simulink model "BMS"  (R2024b)
settings: Solver=ode23tb  StartTime=0.0  StopTime=1  RelTol=1e-3  EnableMultiTasking=on
PreLoadFcn:
  | % Data of Solar Panel
  | %5000[W]/130[W]
  | % Total power generated by solar panel reaches 5[KW].
  | % each solar panel generates power 130[kW].
  | V = [0    40 80 120 160 180 200 217 240 260 280];
  | I = 5000/130*[0.68 0.675 0.67 0.665 0.660 0.655 0.640 0.6 0.48 0.28 0];
  | 
  | %subplot(211);plot(V,I);xlabel('Voltage[V]');ylabel('Current[a]')
  | %subplot(212);plot(V.*I);title('Power[W]')
  | 
  | % Sample Time[s]
  | Ts =5e-6;
  | 
  | 
  | %MPPT + PV Control
  | % PI control pamameter of Voltage control(Outer loop)
  | Kp_V = 50e-3;
  | Ki_V = 10;
  | 
  | % PI Control pamameter of Current control(Inner loop)
  | Kp_I = 25e-3;
  | Ki_I = 10;
  | 
  | % Utility Interconnection Control
  | % PI Control pamameter of Voltage control(Outer loop)
  | Kp_V2 = 0.01;
  | Ki_V2 = 25;
  | 
  | % PI control pamameter of Current control(Inner loop)
  | Kp_I2 = 0.01;
  | Ki_I2 = 25;
  | 
  | 
  | % Difference of voltege using in MPPT
  | dV = 0.5;
  | 
  | % Battery Control
  | % PI Control pamameter of Voltage control(Outer loop)
  | Kp_VB = 0.4;
  | Ki_VB = 2;
  | 
  | % PI control pamameter of Current control(Inner loop)
  | Kp_IB = 0.1;
  | Ki_IB = 0.5;
undefined symbols (not defined in the file): Acid, Ion, Lead, Lithium, sigbuilder_block
libraries: spsBreakerLib x120, spsBatteryLib x111, spsSeriesRLCBranchLib x59, spsVoltageMeasurementLib x17, spsIdealSwitchLib x15, spsMosfetLib x11, slpidlib x9, spsCurrentMeasurementLib x7, spsPWMGeneratorDCDCLib x7, spsDiodeLib x6, spsPWMGenerator2LevelLib x5, spspowerguiLib x3
(part 3 of 6)

== system BMS/Subsystem18/Subsystem7 ==
  Battery : spsBatteryLib/Battery  BatType=Lithium-Ion  NomV=12  NomQ=10  SOC=95  Batt_Tr=30  PresetModel=on  MaxQ=10  MinV=9  FullV=13.9678  Dis_rate=4.3478  R=0.012  Normal_OP=9.0435  expZone="[12.9646     0.491304]"
  Breaker{,1..3} (4 alike) : spsBreakerLib/Breaker  InitialState=0  SwitchingTimes="[1/60  5/60]"  External=on  BreakerResistance=0.01  SnubberResistance=1e6  SnubberCapacitance=inf  Measurements=None  MoreParameters=on  NoBreakLoop=off
  Bus Selector : BusSelector  OutputSignals=SOC (%),Current (A),Voltage (V)
  Scope : Scope  NumInputPorts=3
  Series RLC Branch : spsSeriesRLCBranchLib/Series RLC Branch  LConnTagsString=__new0  RConnTagsString=__new0  BranchType=R  Resistance=1  Inductance=1e-3  SetiL0=off  InitialCurrent=0  Capacitance=1e-6  Setx0=off  InitialVoltage=0  Measurements=None
  + : PMIOPort  Side=Right
  - : PMIOPort  Port=2  Side=Right
  tag scope: s11=global
  wires:
  Battery/1 -> Bus Selector/1
  [c11] -> Breaker3/1, Breaker/1
  Bus Selector/2 -> Scope/2  "<Current (A)>"
  [d11] -> Breaker1/1, Breaker2/1
  Bus Selector/3 -> Scope/3  "<Voltage (V)>"
  Bus Selector/1 -> [s11], Scope/1  "<SOC (%)>"
  connections:
  Breaker2/LConn1 -- Breaker3/RConn1 -- Battery/LConn2
  Breaker1/LConn1 -- Battery/LConn1 -- Breaker/RConn1
  +/RConn1 -- Breaker/LConn1
  Series RLC Branch/LConn1 -- Breaker2/RConn1
  Series RLC Branch/RConn1 -- Breaker1/RConn1
  -/RConn1 -- Breaker3/LConn1

== system BMS/Subsystem18/Subsystem8 ==
  Battery : spsBatteryLib/Battery  BatType=Lithium-Ion  NomV=12  NomQ=10  SOC=95  Batt_Tr=30  PresetModel=on  MaxQ=10  MinV=9  FullV=13.9678  Dis_rate=4.3478  R=0.012  Normal_OP=9.0435  expZone="[12.9646     0.491304]"
  Breaker{,1..3} (4 alike) : spsBreakerLib/Breaker  InitialState=0  SwitchingTimes="[1/60  5/60]"  External=on  BreakerResistance=0.01  SnubberResistance=1e6  SnubberCapacitance=inf  Measurements=None  MoreParameters=on  NoBreakLoop=off
  Bus Selector : BusSelector  OutputSignals=SOC (%),Current (A),Voltage (V)
  Scope : Scope  NumInputPorts=3
  Series RLC Branch : spsSeriesRLCBranchLib/Series RLC Branch  LConnTagsString=__new0  RConnTagsString=__new0  BranchType=R  Resistance=1  Inductance=1e-3  SetiL0=off  InitialCurrent=0  Capacitance=1e-6  Setx0=off  InitialVoltage=0  Measurements=None
  + : PMIOPort  Side=Right
  - : PMIOPort  Port=2  Side=Right
  tag scope: s19=global
  wires:
  Battery/1 -> Bus Selector/1
  [c19] -> Breaker3/1, Breaker/1
  Bus Selector/2 -> Scope/2  "<Current (A)>"
  [d19] -> Breaker1/1, Breaker2/1
  Bus Selector/3 -> Scope/3  "<Voltage (V)>"
  Bus Selector/1 -> [s19], Scope/1  "<SOC (%)>"
  connections:
  Breaker2/LConn1 -- Breaker3/RConn1 -- Battery/LConn2
  Breaker1/LConn1 -- Battery/LConn1 -- Breaker/RConn1
  +/RConn1 -- Breaker/LConn1
  Series RLC Branch/LConn1 -- Breaker2/RConn1
  Series RLC Branch/RConn1 -- Breaker1/RConn1
  -/RConn1 -- Breaker3/LConn1

== system BMS/Subsystem18/Subsystem9 ==
  Battery : spsBatteryLib/Battery  BatType=Lithium-Ion  NomV=12  NomQ=10  SOC=95  Batt_Tr=30  PresetModel=on  MaxQ=10  MinV=9  FullV=13.9678  Dis_rate=4.3478  R=0.012  Normal_OP=9.0435  expZone="[12.9646     0.491304]"
  Breaker{,1..3} (4 alike) : spsBreakerLib/Breaker  InitialState=0  SwitchingTimes="[1/60  5/60]"  External=on  BreakerResistance=0.01  SnubberResistance=1e6  SnubberCapacitance=inf  Measurements=None  MoreParameters=on  NoBreakLoop=off
  Bus Selector : BusSelector  OutputSignals=SOC (%),Current (A),Voltage (V)
  Scope : Scope  NumInputPorts=3
  Series RLC Branch : spsSeriesRLCBranchLib/Series RLC Branch  LConnTagsString=__new0  RConnTagsString=__new0  BranchType=R  Resistance=1  Inductance=1e-3  SetiL0=off  InitialCurrent=0  Capacitance=1e-6  Setx0=off  InitialVoltage=0  Measurements=None
  + : PMIOPort  Side=Right
  - : PMIOPort  Port=2  Side=Right
  tag scope: s20=global
  wires:
  Battery/1 -> Bus Selector/1
  [c20] -> Breaker3/1, Breaker/1
  Bus Selector/2 -> Scope/2  "<Current (A)>"
  [d20] -> Breaker1/1, Breaker2/1
  Bus Selector/3 -> Scope/3  "<Voltage (V)>"
  Bus Selector/1 -> [s20], Scope/1  "<SOC (%)>"
  connections:
  Breaker2/LConn1 -- Breaker3/RConn1 -- Battery/LConn2
  Breaker1/LConn1 -- Battery/LConn1 -- Breaker/RConn1
  +/RConn1 -- Breaker/LConn1
  Series RLC Branch/LConn1 -- Breaker2/RConn1
  Series RLC Branch/RConn1 -- Breaker1/RConn1
  -/RConn1 -- Breaker3/LConn1

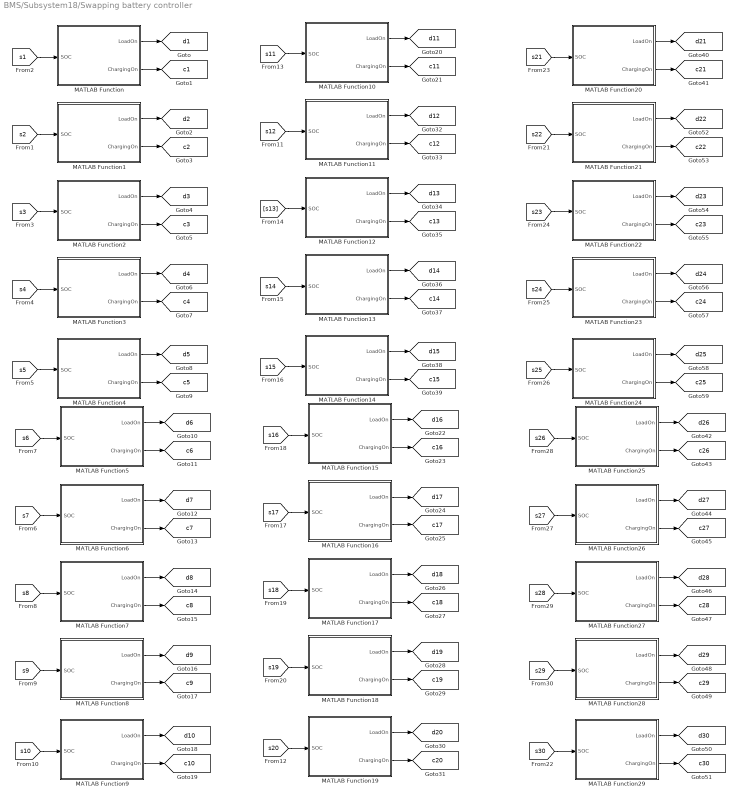
== system BMS/Subsystem18/Swapping battery controller ==
  MATLAB Function : MATLAB Function  TreatAsAtomicUnit=on
  MATLAB Function1 : MATLAB Function  TreatAsAtomicUnit=on
  MATLAB Function10 : MATLAB Function  TreatAsAtomicUnit=on
  MATLAB Function11 : MATLAB Function  TreatAsAtomicUnit=on
  MATLAB Function12 : MATLAB Function  TreatAsAtomicUnit=on
  MATLAB Function13 : MATLAB Function  TreatAsAtomicUnit=on
  MATLAB Function14 : MATLAB Function  TreatAsAtomicUnit=on
  MATLAB Function15 : MATLAB Function  TreatAsAtomicUnit=on
  MATLAB Function16 : MATLAB Function  TreatAsAtomicUnit=on
  MATLAB Function17 : MATLAB Function  TreatAsAtomicUnit=on
  MATLAB Function18 : MATLAB Function  TreatAsAtomicUnit=on
  MATLAB Function19 : MATLAB Function  TreatAsAtomicUnit=on
  MATLAB Function2 : MATLAB Function  TreatAsAtomicUnit=on
  MATLAB Function20 : MATLAB Function  TreatAsAtomicUnit=on
  MATLAB Function21 : MATLAB Function  TreatAsAtomicUnit=on
  MATLAB Function22 : MATLAB Function  TreatAsAtomicUnit=on
  MATLAB Function23 : MATLAB Function  TreatAsAtomicUnit=on
  MATLAB Function24 : MATLAB Function  TreatAsAtomicUnit=on
  MATLAB Function25 : MATLAB Function  TreatAsAtomicUnit=on
  MATLAB Function26 : MATLAB Function  TreatAsAtomicUnit=on
  MATLAB Function27 : MATLAB Function  TreatAsAtomicUnit=on
  MATLAB Function28 : MATLAB Function  TreatAsAtomicUnit=on
  MATLAB Function29 : MATLAB Function  TreatAsAtomicUnit=on
  MATLAB Function3 : MATLAB Function  TreatAsAtomicUnit=on
  MATLAB Function4 : MATLAB Function  TreatAsAtomicUnit=on
  MATLAB Function5 : MATLAB Function  TreatAsAtomicUnit=on
  MATLAB Function6 : MATLAB Function  TreatAsAtomicUnit=on
  MATLAB Function7 : MATLAB Function  TreatAsAtomicUnit=on
  MATLAB Function8 : MATLAB Function  TreatAsAtomicUnit=on
  MATLAB Function9 : MATLAB Function  TreatAsAtomicUnit=on
  tag scope: c10=global, c11=global, c12=global, c13=global, c14=global, c15=global, c16=global, c17=global, c18=global, c19=global, c1=global, c20=global, c21=global, c22=global, c23=global, c24=global, c25=global, c26=global, c27=global, c28=global, c29=global, c2=global, c30=global, c3=global, c4=global, c5=global, c6=global, c7=global, c8=global, c9=global, d10=global, d11=global, d12=global, d13=global, d14=global, d15=global, d16=global, d17=global, d18=global, d19=global, d1=global, d20=global, d21=global, d22=global, d23=global, d24=global, d25=global, d26=global, d27=global, d28=global, d29=global, d2=global, d30=global, d3=global, d4=global, d5=global, d6=global, d7=global, d8=global, d9=global
  wires:
  MATLAB Function10/1(LoadOn) -> [d11]
  MATLAB Function1/2(ChargingOn) -> [c2]
  [s20] -> MATLAB Function19/1(SOC)
  [s22] -> MATLAB Function21/1(SOC)
  MATLAB Function5/1(LoadOn) -> [d6]
  [s16] -> MATLAB Function15/1(SOC)
  [s5] -> MATLAB Function4/1(SOC)
  MATLAB Function/2(ChargingOn) -> [c1]
  MATLAB Function2/2(ChargingOn) -> [c3]
  MATLAB Function26/1(LoadOn) -> [d27]
  [s21] -> MATLAB Function20/1(SOC)
  MATLAB Function18/1(LoadOn) -> [d19]
  MATLAB Function7/2(ChargingOn) -> [c8]
  MATLAB Function12/2(ChargingOn) -> [c13]
  MATLAB Function28/1(LoadOn) -> [d29]
  MATLAB Function4/2(ChargingOn) -> [c5]
  MATLAB Function25/2(ChargingOn) -> [c26]
  [s1] -> MATLAB Function/1(SOC)
  MATLAB Function11/2(ChargingOn) -> [c12]
  MATLAB Function/1(LoadOn) -> [d1]
  MATLAB Function16/1(LoadOn) -> [d17]
  MATLAB Function10/2(ChargingOn) -> [c11]
  [s15] -> MATLAB Function14/1(SOC)
  [s12] -> MATLAB Function11/1(SOC)
  [s3] -> MATLAB Function2/1(SOC)
  MATLAB Function2/1(LoadOn) -> [d3]
  MATLAB Function17/1(LoadOn) -> [d18]
  MATLAB Function13/2(ChargingOn) -> [c14]
  MATLAB Function4/1(LoadOn) -> [d5]
  MATLAB Function14/2(ChargingOn) -> [c15]
  MATLAB Function3/1(LoadOn) -> [d4]
  MATLAB Function6/2(ChargingOn) -> [c7]
  [s7] -> MATLAB Function6/1(SOC)
  MATLAB Function15/1(LoadOn) -> [d16]
  MATLAB Function26/2(ChargingOn) -> [c27]
  [s8] -> MATLAB Function7/1(SOC)
  MATLAB Function6/1(LoadOn) -> [d7]
  MATLAB Function13/1(LoadOn) -> [d14]
  MATLAB Function16/2(ChargingOn) -> [c17]
  MATLAB Function18/2(ChargingOn) -> [c19]
  MATLAB Function5/2(ChargingOn) -> [c6]
  [s6] -> MATLAB Function5/1(SOC)
  [s18] -> MATLAB Function17/1(SOC)
  [s13] -> MATLAB Function12/1(SOC)
  MATLAB Function19/2(ChargingOn) -> [c20]
  MATLAB Function22/1(LoadOn) -> [d23]
  [s27] -> MATLAB Function26/1(SOC)
  MATLAB Function19/1(LoadOn) -> [d20]
  [s26] -> MATLAB Function25/1(SOC)
  [s29] -> MATLAB Function28/1(SOC)
  MATLAB Function8/2(ChargingOn) -> [c9]
  [s17] -> MATLAB Function16/1(SOC)
  MATLAB Function17/2(ChargingOn) -> [c18]
  [s19] -> MATLAB Function18/1(SOC)
  MATLAB Function3/2(ChargingOn) -> [c4]
  MATLAB Function11/1(LoadOn) -> [d12]
  [s11] -> MATLAB Function10/1(SOC)
  MATLAB Function8/1(LoadOn) -> [d9]
  [s2] -> MATLAB Function1/1(SOC)
  MATLAB Function12/1(LoadOn) -> [d13]
  [s10] -> MATLAB Function9/1(SOC)
  MATLAB Function14/1(LoadOn) -> [d15]
  [s14] -> MATLAB Function13/1(SOC)
  MATLAB Function1/1(LoadOn) -> [d2]
  [s4] -> MATLAB Function3/1(SOC)
  MATLAB Function15/2(ChargingOn) -> [c16]
  MATLAB Function7/1(LoadOn) -> [d8]
  [s9] -> MATLAB Function8/1(SOC)
  MATLAB Function9/1(LoadOn) -> [d10]
  MATLAB Function9/2(ChargingOn) -> [c10]
  MATLAB Function29/2(ChargingOn) -> [c30]
  MATLAB Function29/1(LoadOn) -> [d30]
  MATLAB Function27/2(ChargingOn) -> [c28]
  MATLAB Function25/1(LoadOn) -> [d26]
  [s28] -> MATLAB Function27/1(SOC)
  [s30] -> MATLAB Function29/1(SOC)
  MATLAB Function28/2(ChargingOn) -> [c29]
  MATLAB Function23/1(LoadOn) -> [d24]
  [s24] -> MATLAB Function23/1(SOC)
  MATLAB Function23/2(ChargingOn) -> [c24]
  MATLAB Function21/1(LoadOn) -> [d22]
  MATLAB Function27/1(LoadOn) -> [d28]
  MATLAB Function24/1(LoadOn) -> [d25]
  MATLAB Function22/2(ChargingOn) -> [c23]
  [s23] -> MATLAB Function22/1(SOC)
  MATLAB Function24/2(ChargingOn) -> [c25]
  [s25] -> MATLAB Function24/1(SOC)
  MATLAB Function20/2(ChargingOn) -> [c21]
  MATLAB Function21/2(ChargingOn) -> [c22]
  MATLAB Function20/1(LoadOn) -> [d21]

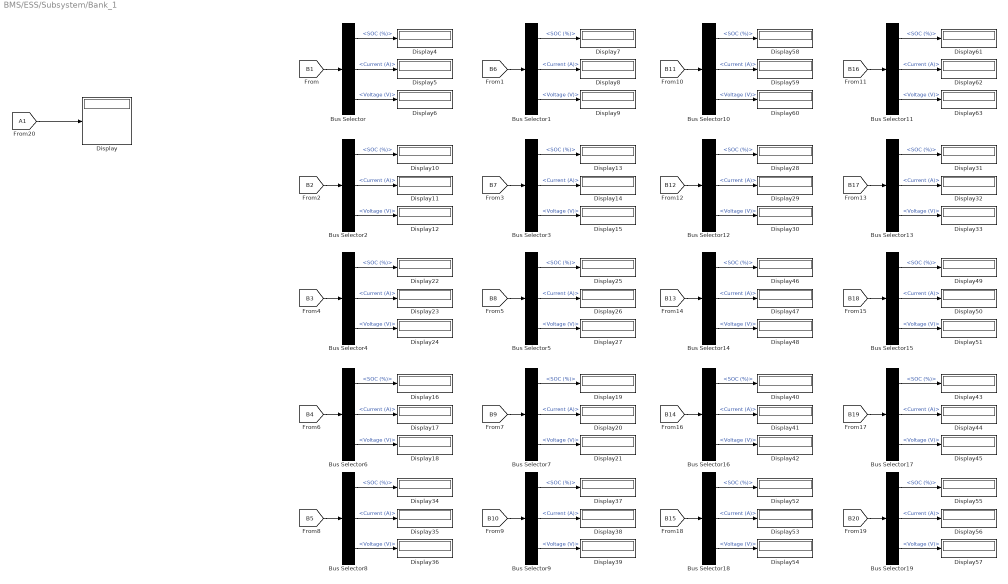
== system BMS/ESS/Subsystem/Bank_1 ==
  Bus Selector{,1..19} (20 alike) : BusSelector  OutputSignals=SOC (%),Current (A),Voltage (V)
  Display{,4..63} (61 alike) : Display
  wires:
  Bus Selector10/3 -> Display60/1  "<Voltage (V)>"
  Bus Selector4/2 -> Display23/1  "<Current (A)>"
  [B9] -> Bus Selector7/1
  Bus Selector7/3 -> Display21/1  "<Voltage (V)>"
  Bus Selector1/1 -> Display7/1  "<SOC (%)>"
  [B7] -> Bus Selector3/1
  Bus Selector16/3 -> Display42/1  "<Voltage (V)>"
  [B8] -> Bus Selector5/1
  Bus Selector17/1 -> Display43/1  "<SOC (%)>"
  Bus Selector1/2 -> Display8/1  "<Current (A)>"
  Bus Selector/3 -> Display6/1  "<Voltage (V)>"
  Bus Selector4/3 -> Display24/1  "<Voltage (V)>"
  [B4] -> Bus Selector6/1
  Bus Selector18/3 -> Display54/1  "<Voltage (V)>"
  [B19] -> Bus Selector17/1
  Bus Selector6/2 -> Display17/1  "<Current (A)>"
  Bus Selector/2 -> Display5/1  "<Current (A)>"
  [B3] -> Bus Selector4/1
  [B6] -> Bus Selector1/1
  Bus Selector12/3 -> Display30/1  "<Voltage (V)>"
  Bus Selector10/1 -> Display58/1  "<SOC (%)>"
  Bus Selector7/2 -> Display20/1  "<Current (A)>"
  Bus Selector6/1 -> Display16/1  "<SOC (%)>"
  Bus Selector16/2 -> Display41/1  "<Current (A)>"
  Bus Selector11/1 -> Display61/1  "<SOC (%)>"
  Bus Selector9/3 -> Display39/1  "<Voltage (V)>"
  Bus Selector3/2 -> Display14/1  "<Current (A)>"
  [B20] -> Bus Selector19/1
  Bus Selector5/2 -> Display26/1  "<Current (A)>"
  Bus Selector5/1 -> Display25/1  "<SOC (%)>"
  Bus Selector7/1 -> Display19/1  "<SOC (%)>"
  Bus Selector5/3 -> Display27/1  "<Voltage (V)>"
  Bus Selector4/1 -> Display22/1  "<SOC (%)>"
  Bus Selector9/1 -> Display37/1  "<SOC (%)>"
  Bus Selector2/3 -> Display12/1  "<Voltage (V)>"
  Bus Selector6/3 -> Display18/1  "<Voltage (V)>"
  [B17] -> Bus Selector13/1
  Bus Selector/1 -> Display4/1  "<SOC (%)>"
  Bus Selector1/3 -> Display9/1  "<Voltage (V)>"
  Bus Selector9/2 -> Display38/1  "<Current (A)>"
  Bus Selector17/2 -> Display44/1  "<Current (A)>"
  [B10] -> Bus Selector9/1
  Bus Selector8/1 -> Display34/1  "<SOC (%)>"
  Bus Selector11/3 -> Display63/1  "<Voltage (V)>"
  Bus Selector8/2 -> Display35/1  "<Current (A)>"
  Bus Selector8/3 -> Display36/1  "<Voltage (V)>"
  [B12] -> Bus Selector12/1
  [B2] -> Bus Selector2/1
  [B5] -> Bus Selector8/1
  Bus Selector2/2 -> Display11/1  "<Current (A)>"
  Bus Selector19/3 -> Display57/1  "<Voltage (V)>"
  Bus Selector3/3 -> Display15/1  "<Voltage (V)>"
  Bus Selector3/1 -> Display13/1  "<SOC (%)>"
  Bus Selector15/3 -> Display51/1  "<Voltage (V)>"
  [B11] -> Bus Selector10/1
  Bus Selector13/2 -> Display32/1  "<Current (A)>"
  [B15] -> Bus Selector18/1
  Bus Selector2/1 -> Display10/1  "<SOC (%)>"
  Bus Selector19/2 -> Display56/1  "<Current (A)>"
  [B1] -> Bus Selector/1
  Bus Selector12/1 -> Display28/1  "<SOC (%)>"
  Bus Selector12/2 -> Display29/1  "<Current (A)>"
  Bus Selector19/1 -> Display55/1  "<SOC (%)>"
  Bus Selector13/3 -> Display33/1  "<Voltage (V)>"
  Bus Selector13/1 -> Display31/1  "<SOC (%)>"
  Bus Selector18/1 -> Display52/1  "<SOC (%)>"
  Bus Selector18/2 -> Display53/1  "<Current (A)>"
  Bus Selector11/2 -> Display62/1  "<Current (A)>"
  Bus Selector15/1 -> Display49/1  "<SOC (%)>"
  Bus Selector14/1 -> Display46/1  "<SOC (%)>"
  Bus Selector14/3 -> Display48/1  "<Voltage (V)>"
  [B16] -> Bus Selector11/1
  Bus Selector15/2 -> Display50/1  "<Current (A)>"
  Bus Selector10/2 -> Display59/1  "<Current (A)>"
  [B14] -> Bus Selector16/1
  Bus Selector16/1 -> Display40/1  "<SOC (%)>"
  [B18] -> Bus Selector15/1
  [B13] -> Bus Selector14/1
  Bus Selector17/3 -> Display45/1  "<Voltage (V)>"
  Bus Selector14/2 -> Display47/1  "<Current (A)>"
  [A1] -> Display/1

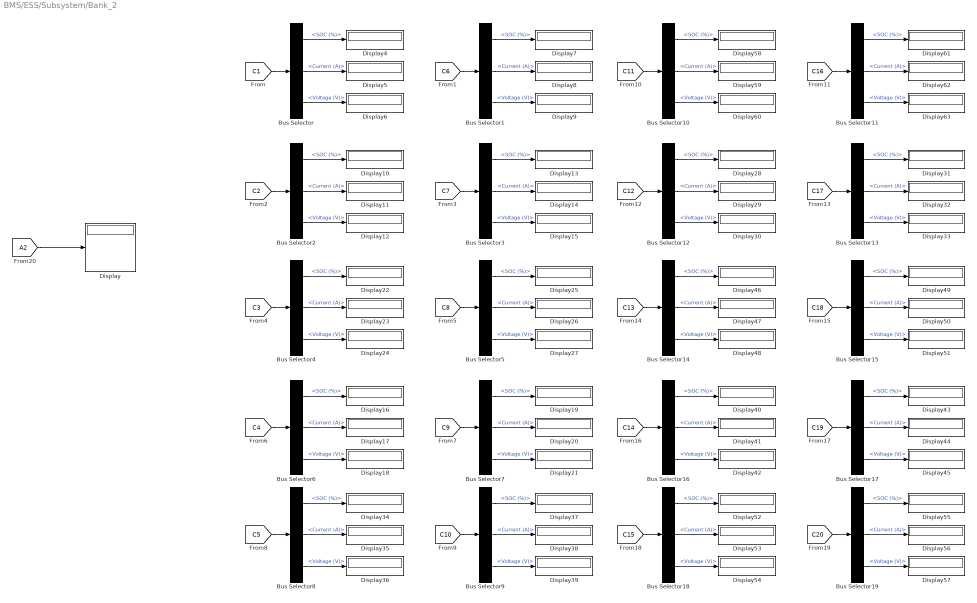
== system BMS/ESS/Subsystem/Bank_2 ==
  Bus Selector{,1..19} (20 alike) : BusSelector  OutputSignals=SOC (%),Current (A),Voltage (V)
  Display{,4..63} (61 alike) : Display
  wires:
  Bus Selector10/3 -> Display60/1  "<Voltage (V)>"
  Bus Selector4/2 -> Display23/1  "<Current (A)>"
  [C9] -> Bus Selector7/1
  Bus Selector7/3 -> Display21/1  "<Voltage (V)>"
  Bus Selector1/1 -> Display7/1  "<SOC (%)>"
  [C7] -> Bus Selector3/1
  Bus Selector16/3 -> Display42/1  "<Voltage (V)>"
  [C8] -> Bus Selector5/1
  Bus Selector17/1 -> Display43/1  "<SOC (%)>"
  Bus Selector1/2 -> Display8/1  "<Current (A)>"
  Bus Selector/3 -> Display6/1  "<Voltage (V)>"
  Bus Selector4/3 -> Display24/1  "<Voltage (V)>"
  [C4] -> Bus Selector6/1
  Bus Selector18/3 -> Display54/1  "<Voltage (V)>"
  [C19] -> Bus Selector17/1
  Bus Selector6/2 -> Display17/1  "<Current (A)>"
  Bus Selector/2 -> Display5/1  "<Current (A)>"
  [C3] -> Bus Selector4/1
  [C6] -> Bus Selector1/1
  Bus Selector12/3 -> Display30/1  "<Voltage (V)>"
  Bus Selector10/1 -> Display58/1  "<SOC (%)>"
  Bus Selector7/2 -> Display20/1  "<Current (A)>"
  Bus Selector6/1 -> Display16/1  "<SOC (%)>"
  Bus Selector16/2 -> Display41/1  "<Current (A)>"
  Bus Selector11/1 -> Display61/1  "<SOC (%)>"
  Bus Selector9/3 -> Display39/1  "<Voltage (V)>"
  Bus Selector3/2 -> Display14/1  "<Current (A)>"
  [C20] -> Bus Selector19/1
  Bus Selector5/2 -> Display26/1  "<Current (A)>"
  Bus Selector5/1 -> Display25/1  "<SOC (%)>"
  Bus Selector7/1 -> Display19/1  "<SOC (%)>"
  Bus Selector5/3 -> Display27/1  "<Voltage (V)>"
  Bus Selector4/1 -> Display22/1  "<SOC (%)>"
  Bus Selector9/1 -> Display37/1  "<SOC (%)>"
  Bus Selector2/3 -> Display12/1  "<Voltage (V)>"
  Bus Selector6/3 -> Display18/1  "<Voltage (V)>"
  [C17] -> Bus Selector13/1
  Bus Selector/1 -> Display4/1  "<SOC (%)>"
  Bus Selector1/3 -> Display9/1  "<Voltage (V)>"
  Bus Selector9/2 -> Display38/1  "<Current (A)>"
  Bus Selector17/2 -> Display44/1  "<Current (A)>"
  [C10] -> Bus Selector9/1
  Bus Selector8/1 -> Display34/1  "<SOC (%)>"
  Bus Selector11/3 -> Display63/1  "<Voltage (V)>"
  Bus Selector8/2 -> Display35/1  "<Current (A)>"
  Bus Selector8/3 -> Display36/1  "<Voltage (V)>"
  [C12] -> Bus Selector12/1
  [C2] -> Bus Selector2/1
  [C5] -> Bus Selector8/1
  Bus Selector2/2 -> Display11/1  "<Current (A)>"
  Bus Selector19/3 -> Display57/1  "<Voltage (V)>"
  Bus Selector3/3 -> Display15/1  "<Voltage (V)>"
  Bus Selector3/1 -> Display13/1  "<SOC (%)>"
  Bus Selector15/3 -> Display51/1  "<Voltage (V)>"
  [C11] -> Bus Selector10/1
  Bus Selector13/2 -> Display32/1  "<Current (A)>"
  [C15] -> Bus Selector18/1
  Bus Selector2/1 -> Display10/1  "<SOC (%)>"
  Bus Selector19/2 -> Display56/1  "<Current (A)>"
  [C1] -> Bus Selector/1
  Bus Selector12/1 -> Display28/1  "<SOC (%)>"
  Bus Selector12/2 -> Display29/1  "<Current (A)>"
  Bus Selector19/1 -> Display55/1  "<SOC (%)>"
  Bus Selector13/3 -> Display33/1  "<Voltage (V)>"
  Bus Selector13/1 -> Display31/1  "<SOC (%)>"
  Bus Selector18/1 -> Display52/1  "<SOC (%)>"
  Bus Selector18/2 -> Display53/1  "<Current (A)>"
  Bus Selector11/2 -> Display62/1  "<Current (A)>"
  Bus Selector15/1 -> Display49/1  "<SOC (%)>"
  Bus Selector14/1 -> Display46/1  "<SOC (%)>"
  Bus Selector14/3 -> Display48/1  "<Voltage (V)>"
  [C16] -> Bus Selector11/1
  Bus Selector15/2 -> Display50/1  "<Current (A)>"
  Bus Selector10/2 -> Display59/1  "<Current (A)>"
  [C14] -> Bus Selector16/1
  Bus Selector16/1 -> Display40/1  "<SOC (%)>"
  [C18] -> Bus Selector15/1
  [C13] -> Bus Selector14/1
  Bus Selector17/3 -> Display45/1  "<Voltage (V)>"
  Bus Selector14/2 -> Display47/1  "<Current (A)>"
  [A2] -> Display/1

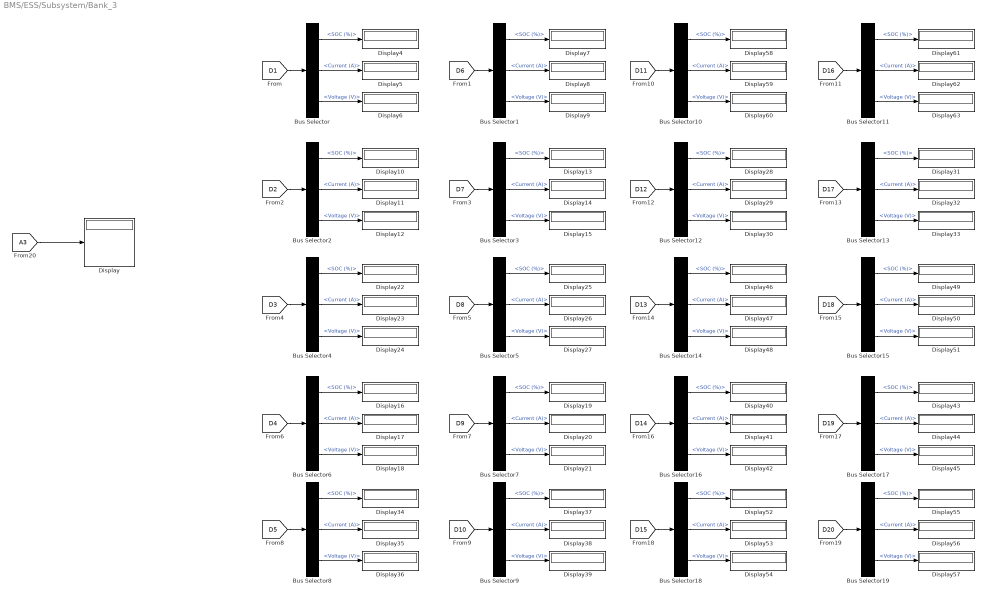
== system BMS/ESS/Subsystem/Bank_3 ==
  Bus Selector{,1..19} (20 alike) : BusSelector  OutputSignals=SOC (%),Current (A),Voltage (V)
  Display{,4..63} (61 alike) : Display
  wires:
  Bus Selector10/3 -> Display60/1  "<Voltage (V)>"
  Bus Selector4/2 -> Display23/1  "<Current (A)>"
  [D9] -> Bus Selector7/1
  Bus Selector7/3 -> Display21/1  "<Voltage (V)>"
  Bus Selector1/1 -> Display7/1  "<SOC (%)>"
  [D7] -> Bus Selector3/1
  Bus Selector16/3 -> Display42/1  "<Voltage (V)>"
  [D8] -> Bus Selector5/1
  Bus Selector17/1 -> Display43/1  "<SOC (%)>"
  Bus Selector1/2 -> Display8/1  "<Current (A)>"
  Bus Selector/3 -> Display6/1  "<Voltage (V)>"
  Bus Selector4/3 -> Display24/1  "<Voltage (V)>"
  [D4] -> Bus Selector6/1
  Bus Selector18/3 -> Display54/1  "<Voltage (V)>"
  [D19] -> Bus Selector17/1
  Bus Selector6/2 -> Display17/1  "<Current (A)>"
  Bus Selector/2 -> Display5/1  "<Current (A)>"
  [D3] -> Bus Selector4/1
  [D6] -> Bus Selector1/1
  Bus Selector12/3 -> Display30/1  "<Voltage (V)>"
  Bus Selector10/1 -> Display58/1  "<SOC (%)>"
  Bus Selector7/2 -> Display20/1  "<Current (A)>"
  Bus Selector6/1 -> Display16/1  "<SOC (%)>"
  Bus Selector16/2 -> Display41/1  "<Current (A)>"
  Bus Selector11/1 -> Display61/1  "<SOC (%)>"
  Bus Selector9/3 -> Display39/1  "<Voltage (V)>"
  Bus Selector3/2 -> Display14/1  "<Current (A)>"
  [D20] -> Bus Selector19/1
  Bus Selector5/2 -> Display26/1  "<Current (A)>"
  Bus Selector5/1 -> Display25/1  "<SOC (%)>"
  Bus Selector7/1 -> Display19/1  "<SOC (%)>"
  Bus Selector5/3 -> Display27/1  "<Voltage (V)>"
  Bus Selector4/1 -> Display22/1  "<SOC (%)>"
  Bus Selector9/1 -> Display37/1  "<SOC (%)>"
  Bus Selector2/3 -> Display12/1  "<Voltage (V)>"
  Bus Selector6/3 -> Display18/1  "<Voltage (V)>"
  [D17] -> Bus Selector13/1
  Bus Selector/1 -> Display4/1  "<SOC (%)>"
  Bus Selector1/3 -> Display9/1  "<Voltage (V)>"
  Bus Selector9/2 -> Display38/1  "<Current (A)>"
  Bus Selector17/2 -> Display44/1  "<Current (A)>"
  [D10] -> Bus Selector9/1
  Bus Selector8/1 -> Display34/1  "<SOC (%)>"
  Bus Selector11/3 -> Display63/1  "<Voltage (V)>"
  Bus Selector8/2 -> Display35/1  "<Current (A)>"
  Bus Selector8/3 -> Display36/1  "<Voltage (V)>"
  [D12] -> Bus Selector12/1
  [D2] -> Bus Selector2/1
  [D5] -> Bus Selector8/1
  Bus Selector2/2 -> Display11/1  "<Current (A)>"
  Bus Selector19/3 -> Display57/1  "<Voltage (V)>"
  Bus Selector3/3 -> Display15/1  "<Voltage (V)>"
  Bus Selector3/1 -> Display13/1  "<SOC (%)>"
  Bus Selector15/3 -> Display51/1  "<Voltage (V)>"
  [D11] -> Bus Selector10/1
  Bus Selector13/2 -> Display32/1  "<Current (A)>"
  [D15] -> Bus Selector18/1
  Bus Selector2/1 -> Display10/1  "<SOC (%)>"
  Bus Selector19/2 -> Display56/1  "<Current (A)>"
  [D1] -> Bus Selector/1
  Bus Selector12/1 -> Display28/1  "<SOC (%)>"
  Bus Selector12/2 -> Display29/1  "<Current (A)>"
  Bus Selector19/1 -> Display55/1  "<SOC (%)>"
  Bus Selector13/3 -> Display33/1  "<Voltage (V)>"
  Bus Selector13/1 -> Display31/1  "<SOC (%)>"
  Bus Selector18/1 -> Display52/1  "<SOC (%)>"
  Bus Selector18/2 -> Display53/1  "<Current (A)>"
  Bus Selector11/2 -> Display62/1  "<Current (A)>"
  Bus Selector15/1 -> Display49/1  "<SOC (%)>"
  Bus Selector14/1 -> Display46/1  "<SOC (%)>"
  Bus Selector14/3 -> Display48/1  "<Voltage (V)>"
  [D16] -> Bus Selector11/1
  Bus Selector15/2 -> Display50/1  "<Current (A)>"
  Bus Selector10/2 -> Display59/1  "<Current (A)>"
  [D14] -> Bus Selector16/1
  Bus Selector16/1 -> Display40/1  "<SOC (%)>"
  [D18] -> Bus Selector15/1
  [D13] -> Bus Selector14/1
  Bus Selector17/3 -> Display45/1  "<Voltage (V)>"
  Bus Selector14/2 -> Display47/1  "<Current (A)>"
  [A3] -> Display/1

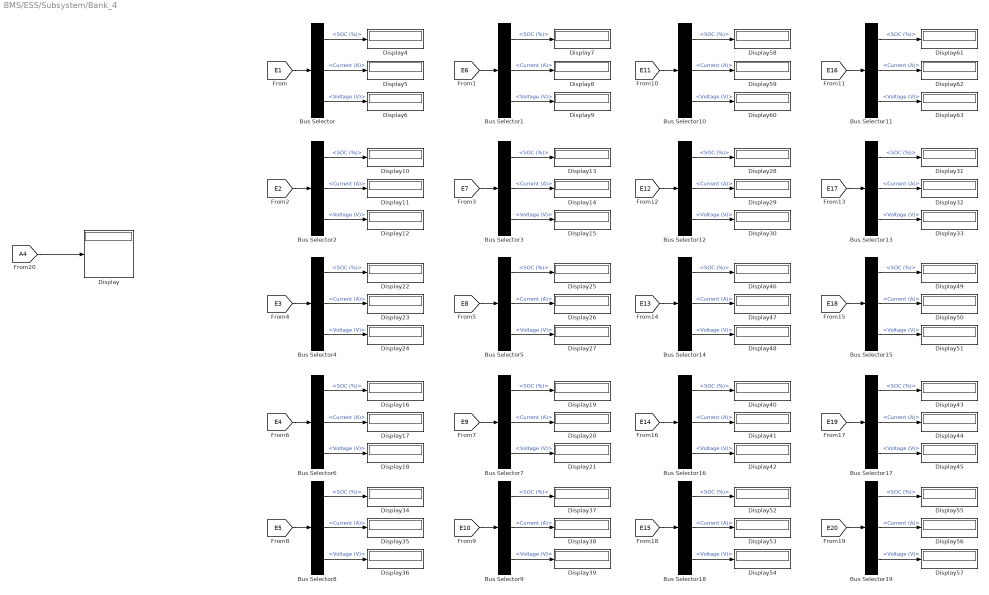
== system BMS/ESS/Subsystem/Bank_4 ==
  Bus Selector{,1..19} (20 alike) : BusSelector  OutputSignals=SOC (%),Current (A),Voltage (V)
  Display{,4..63} (61 alike) : Display
  wires:
  Bus Selector10/3 -> Display60/1  "<Voltage (V)>"
  Bus Selector4/2 -> Display23/1  "<Current (A)>"
  [E9] -> Bus Selector7/1
  Bus Selector7/3 -> Display21/1  "<Voltage (V)>"
  Bus Selector1/1 -> Display7/1  "<SOC (%)>"
  [E7] -> Bus Selector3/1
  Bus Selector16/3 -> Display42/1  "<Voltage (V)>"
  [E8] -> Bus Selector5/1
  Bus Selector17/1 -> Display43/1  "<SOC (%)>"
  Bus Selector1/2 -> Display8/1  "<Current (A)>"
  Bus Selector/3 -> Display6/1  "<Voltage (V)>"
  Bus Selector4/3 -> Display24/1  "<Voltage (V)>"
  [E4] -> Bus Selector6/1
  Bus Selector18/3 -> Display54/1  "<Voltage (V)>"
  [E19] -> Bus Selector17/1
  Bus Selector6/2 -> Display17/1  "<Current (A)>"
  Bus Selector/2 -> Display5/1  "<Current (A)>"
  [E3] -> Bus Selector4/1
  [E6] -> Bus Selector1/1
  Bus Selector12/3 -> Display30/1  "<Voltage (V)>"
  Bus Selector10/1 -> Display58/1  "<SOC (%)>"
  Bus Selector7/2 -> Display20/1  "<Current (A)>"
  Bus Selector6/1 -> Display16/1  "<SOC (%)>"
  Bus Selector16/2 -> Display41/1  "<Current (A)>"
  Bus Selector11/1 -> Display61/1  "<SOC (%)>"
  Bus Selector9/3 -> Display39/1  "<Voltage (V)>"
  Bus Selector3/2 -> Display14/1  "<Current (A)>"
  [E20] -> Bus Selector19/1
  Bus Selector5/2 -> Display26/1  "<Current (A)>"
  Bus Selector5/1 -> Display25/1  "<SOC (%)>"
  Bus Selector7/1 -> Display19/1  "<SOC (%)>"
  Bus Selector5/3 -> Display27/1  "<Voltage (V)>"
  Bus Selector4/1 -> Display22/1  "<SOC (%)>"
  Bus Selector9/1 -> Display37/1  "<SOC (%)>"
  Bus Selector2/3 -> Display12/1  "<Voltage (V)>"
  Bus Selector6/3 -> Display18/1  "<Voltage (V)>"
  [E17] -> Bus Selector13/1
  Bus Selector/1 -> Display4/1  "<SOC (%)>"
  Bus Selector1/3 -> Display9/1  "<Voltage (V)>"
  Bus Selector9/2 -> Display38/1  "<Current (A)>"
  Bus Selector17/2 -> Display44/1  "<Current (A)>"
  [E10] -> Bus Selector9/1
  Bus Selector8/1 -> Display34/1  "<SOC (%)>"
  Bus Selector11/3 -> Display63/1  "<Voltage (V)>"
  Bus Selector8/2 -> Display35/1  "<Current (A)>"
  Bus Selector8/3 -> Display36/1  "<Voltage (V)>"
  [E12] -> Bus Selector12/1
  [E2] -> Bus Selector2/1
  [E5] -> Bus Selector8/1
  Bus Selector2/2 -> Display11/1  "<Current (A)>"
  Bus Selector19/3 -> Display57/1  "<Voltage (V)>"
  Bus Selector3/3 -> Display15/1  "<Voltage (V)>"
  Bus Selector3/1 -> Display13/1  "<SOC (%)>"
  Bus Selector15/3 -> Display51/1  "<Voltage (V)>"
  [E11] -> Bus Selector10/1
  Bus Selector13/2 -> Display32/1  "<Current (A)>"
  [E15] -> Bus Selector18/1
  Bus Selector2/1 -> Display10/1  "<SOC (%)>"
  Bus Selector19/2 -> Display56/1  "<Current (A)>"
  [E1] -> Bus Selector/1
  Bus Selector12/1 -> Display28/1  "<SOC (%)>"
  Bus Selector12/2 -> Display29/1  "<Current (A)>"
  Bus Selector19/1 -> Display55/1  "<SOC (%)>"
  Bus Selector13/3 -> Display33/1  "<Voltage (V)>"
  Bus Selector13/1 -> Display31/1  "<SOC (%)>"
  Bus Selector18/1 -> Display52/1  "<SOC (%)>"
  Bus Selector18/2 -> Display53/1  "<Current (A)>"
  Bus Selector11/2 -> Display62/1  "<Current (A)>"
  Bus Selector15/1 -> Display49/1  "<SOC (%)>"
  Bus Selector14/1 -> Display46/1  "<SOC (%)>"
  Bus Selector14/3 -> Display48/1  "<Voltage (V)>"
  [E16] -> Bus Selector11/1
  Bus Selector15/2 -> Display50/1  "<Current (A)>"
  Bus Selector10/2 -> Display59/1  "<Current (A)>"
  [E14] -> Bus Selector16/1
  Bus Selector16/1 -> Display40/1  "<SOC (%)>"
  [E18] -> Bus Selector15/1
  [E13] -> Bus Selector14/1
  Bus Selector17/3 -> Display45/1  "<Voltage (V)>"
  Bus Selector14/2 -> Display47/1  "<Current (A)>"
  [A4] -> Display/1

== system BMS/ESS/Subsystem/PCC Point of common couppling ==
  note: ESS
  note: Grid
  note: Solar
  note: Solar
  note: Grid
  bank_1 + : PMIOPort  Side=Left
  bank_1 - : PMIOPort  Port=2  Side=Left
  bank_2 + : PMIOPort  Port=3  Side=Left
  bank_3 - : PMIOPort  Port=4  Side=Left
  bank_4 + : PMIOPort  Port=5  Side=Left
  bank_5 + : PMIOPort  Port=6  Side=Left
  bank_4 - : PMIOPort  Port=7  Side=Left
  bank_5 - : PMIOPort  Port=8  Side=Left
  DC + : PMIOPort  Port=9  Side=Right
  DC - : PMIOPort  Port=10  Side=Right
  connections:
  bank_5 +/RConn1 -- bank_1 +/RConn1 -- bank_2 +/RConn1 -- DC +/RConn1 -- bank_4 +/RConn1
  DC -/RConn1 -- bank_1 -/RConn1 -- bank_3 -/RConn1 -- bank_4 -/RConn1 -- bank_5 -/RConn1

== system BMS/Grid1/Wall charger Connection Box/Battery Switching Control ==
  Control : Inport
  Battery : spsBatteryLib/Battery  BatType=Lead-Acid  NomV=400  NomQ=5.4  SOC=100  Batt_Tr=30  PresetModel=on  MaxQ=5.625  MinV=300  FullV=435.5263  Dis_rate=1.08  R=0.74074  Normal_OP=1.6755  expZone="[407.2368         0.018]"
  Ideal Switch{,1,3..4} (4 alike) : spsIdealSwitchLib/Ideal Switch  Ron=0.001  Lon=0  IC=0  Rs=1e5  Cs=inf  Measurements=off
  NOT : Logic  Operator=NOT  IconShape=distinctive  AllPortsSameDT=off  OutDataTypeStr=boolean
  discharge + : PMIOPort  Side=Left
  discharge - : PMIOPort  Port=2  Side=Left
  charge + : PMIOPort  Port=3  Side=Left
  charge - : PMIOPort  Port=4  Side=Left
  battery + : PMIOPort  Port=5  Side=Right
  battery - : PMIOPort  Port=6  Side=Right
  wires:
  Control/1 -> NOT/1, Ideal Switch1/1, Ideal Switch/1
  NOT/1 -> Ideal Switch4/1, Ideal Switch3/1
  connections:
  charge -/RConn1 -- Ideal Switch4/RConn1
  discharge +/RConn1 -- Ideal Switch/RConn1
  battery -/RConn1 -- Battery/LConn2 -- Ideal Switch1/LConn1 -- Ideal Switch4/LConn1
  discharge -/RConn1 -- Ideal Switch1/RConn1
  Ideal Switch/LConn1 -- Battery/LConn1 -- battery +/RConn1 -- Ideal Switch3/LConn1
  charge +/RConn1 -- Ideal Switch3/RConn1

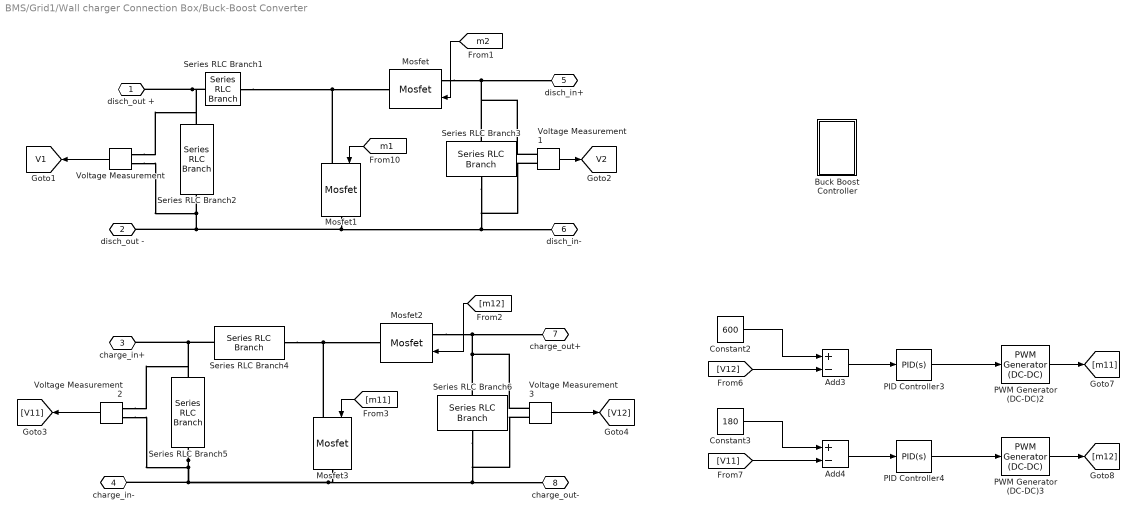
== system BMS/Grid1/Wall charger Connection Box/Buck-Boost Converter ==
  Add3 : Sum  Inputs=+-
  Add4 : Sum  Inputs=+-
  Buck Boost Controller : Subsystem
  Constant2 : Constant  Value=600
  Constant3 : Constant  Value=180
  Mosfet{,1..3} (4 alike) : spsMosfetLib/Mosfet  Ron=0.1  Lon=0  Rd=0.01  Vfd=0  IC=0  Rs=1e5  Cs=inf  Measurements=off
  PID Controller3 : slpidlib/PID Controller  Controller=PID  Form=Parallel  TimeDomain=Continuous-time  UseExternalTs=off  SampleTime=-1  IntegratorMethod=Forward Euler  FilterMethod=Forward Euler  ControllerParametersSource=internal  P=0  I=7  UseKiTs=off  D=0  UseExternalDerivativeSource=off  N=100  UseFilter=on  TunerSelectOption=Transfer Function Based (PID Tuner App)  InitialConditionSource=internal  InitialConditionForIntegrator=0  InitialConditionForFilter=0  DifferentiatorICPrevScaledInput=0  ExternalReset=none  TrackingMode=off  Kt=1  LimitOutput=off  SatLimitsSource=internal  UpperSaturationLimit=inf  LowerSaturationLimit=-inf  LinearizeAsGain=on  AntiWindupMode=none  Kb=1  LimitIntegrator=off  UpperIntegratorSaturationLimit=inf  LowerIntegratorSaturationLimit=-inf  POutMin=[]  POutMax=[]  IOutMin=[]  IOutMax=[]  DOutMin=[]  DOutMax=[]  NOutMin=[]  NOutMax=[]  SumOutMin=[]  SumOutMax=[]  SaturationOutMin=[]  SaturationOutMax=[]  PParamMin=[]  PParamMax=[]  IParamMin=[]  IParamMax=[]  DParamMin=[]  DParamMax=[]  NParamMin=[]  NParamMax=[]  KbParamMin=[]  KbParamMax=[]  KtParamMin=[]  KtParamMax=[]  KbOutMin=[]  KbOutMax=[]  KtOutMin=[]  KtOutMax=[]  IntegratorOutMin=[]  IntegratorOutMax=[]  FilterOutMin=[]  FilterOutMax=[]  SumI1OutMin=[]  SumI1OutMax=[]  SumI2OutMin=[]  SumI2OutMax=[]  SumI3OutMin=[]  SumI3OutMax=[]  SumI4OutMin=[]  SumI4OutMax=[]  SumDOutMin=[]  SumDOutMax=[]  DifferentiatorOutMin=[]  DifferentiatorOutMax=[]  FilterDiffOutCoefMin=[]  FilterDiffOutCoefMax=[]  ReciprocalOutMin=[]  ReciprocalOutMax=[]  SumDenOutMin=[]  SumDenOutMax=[]  SumNumOutMin=[]  SumNumOutMax=[]  DivideOutMin=[]  DivideOutMax=[]  UdiffTsProdOutMin=[]  UdiffTsProdOutMax=[]  NTsProdOutMin=[]  NTsProdOutMax=[]  UintegralTsProdOutMin=[]  UintegralTsProdOutMax=[]  UngainTsProdOutMin=[]  UngainTsProdOutMax=[]  ClampingZeroOutDataTypeStr=Inherit: Inherit via back propagation  ClampingZeroOutMin=[]  ClampingZeroOutMax=[]  FilterDenConstantOutDataTypeStr=Inherit: Inherit via back propagation  FilterDenConstantOutMin=[]  FilterDenConstantOutMax=[]  PCopyOutDataTypeStr=Inherit: Inherit via back propagation  PCopyOutMin=[]  PCopyOutMax=[]  NCopyOutDataTypeStr=Inherit: Inherit via back propagation  NCopyOutMin=[]  NCopyOutMax=[]  IntegratorContinuousStateAttributes=''  IntegratorStateMustResolveToSignalObject=off  IntegratorRTWStateStorageClass=Auto  FilterContinuousStateAttributes=''  FilterStateMustResolveToSignalObject=off  FilterRTWStateStorageClass=Auto  ParallelPVariant=InternalParameters  IdealPVariant=Disabled  IVariant=InternalParameters  DVariant=InternalParameters  IntegratorVariant=Continuous  SatVariant=Disabled  AWVariant=Passthrough  PCopyVariant=Disabled  TRVariant=Disabled  FdbkBlocksVariant=Forward  IdealPFdbkVariant=Disabled  SatFdbkVariant=Disabled  DerivativeFilterVariant=ContFilter  NVariant=InternalParameters  NCopyVariant=Disabled  FilterICVariant=InternalICsFilter  IntegratorICVariant=InternalICs  ExternalResetVariant=Disabled  TRSumVariant=Passthrough  SumFdbkVariant=Disabled  SumVariant=Sum_PID  TsampFilterVariant=InternalTs  TsampNgainVariant=Passthrough  TsampIntegralVariant=Disabled_SignalSpec  ExternalSaturationOutDataTypeStr=Inherit: Same as second input  DerivativeSourceVariant=ErrorSignal  PreIntVariant=InternalPreInt
  PID Controller4 : slpidlib/PID Controller  Controller=PID  Form=Parallel  TimeDomain=Continuous-time  UseExternalTs=off  SampleTime=-1  IntegratorMethod=Forward Euler  FilterMethod=Forward Euler  ControllerParametersSource=internal  P=0  I=7  UseKiTs=off  D=0  UseExternalDerivativeSource=off  N=100  UseFilter=on  TunerSelectOption=Transfer Function Based (PID Tuner App)  InitialConditionSource=internal  InitialConditionForIntegrator=0  InitialConditionForFilter=0  DifferentiatorICPrevScaledInput=0  ExternalReset=none  TrackingMode=off  Kt=1  LimitOutput=off  SatLimitsSource=internal  UpperSaturationLimit=inf  LowerSaturationLimit=-inf  LinearizeAsGain=on  AntiWindupMode=none  Kb=1  LimitIntegrator=off  UpperIntegratorSaturationLimit=inf  LowerIntegratorSaturationLimit=-inf  POutMin=[]  POutMax=[]  IOutMin=[]  IOutMax=[]  DOutMin=[]  DOutMax=[]  NOutMin=[]  NOutMax=[]  SumOutMin=[]  SumOutMax=[]  SaturationOutMin=[]  SaturationOutMax=[]  PParamMin=[]  PParamMax=[]  IParamMin=[]  IParamMax=[]  DParamMin=[]  DParamMax=[]  NParamMin=[]  NParamMax=[]  KbParamMin=[]  KbParamMax=[]  KtParamMin=[]  KtParamMax=[]  KbOutMin=[]  KbOutMax=[]  KtOutMin=[]  KtOutMax=[]  IntegratorOutMin=[]  IntegratorOutMax=[]  FilterOutMin=[]  FilterOutMax=[]  SumI1OutMin=[]  SumI1OutMax=[]  SumI2OutMin=[]  SumI2OutMax=[]  SumI3OutMin=[]  SumI3OutMax=[]  SumI4OutMin=[]  SumI4OutMax=[]  SumDOutMin=[]  SumDOutMax=[]  DifferentiatorOutMin=[]  DifferentiatorOutMax=[]  FilterDiffOutCoefMin=[]  FilterDiffOutCoefMax=[]  ReciprocalOutMin=[]  ReciprocalOutMax=[]  SumDenOutMin=[]  SumDenOutMax=[]  SumNumOutMin=[]  SumNumOutMax=[]  DivideOutMin=[]  DivideOutMax=[]  UdiffTsProdOutMin=[]  UdiffTsProdOutMax=[]  NTsProdOutMin=[]  NTsProdOutMax=[]  UintegralTsProdOutMin=[]  UintegralTsProdOutMax=[]  UngainTsProdOutMin=[]  UngainTsProdOutMax=[]  ClampingZeroOutDataTypeStr=Inherit: Inherit via back propagation  ClampingZeroOutMin=[]  ClampingZeroOutMax=[]  FilterDenConstantOutDataTypeStr=Inherit: Inherit via back propagation  FilterDenConstantOutMin=[]  FilterDenConstantOutMax=[]  PCopyOutDataTypeStr=Inherit: Inherit via back propagation  PCopyOutMin=[]  PCopyOutMax=[]  NCopyOutDataTypeStr=Inherit: Inherit via back propagation  NCopyOutMin=[]  NCopyOutMax=[]  IntegratorContinuousStateAttributes=''  IntegratorStateMustResolveToSignalObject=off  IntegratorRTWStateStorageClass=Auto  FilterContinuousStateAttributes=''  FilterStateMustResolveToSignalObject=off  FilterRTWStateStorageClass=Auto  ParallelPVariant=InternalParameters  IdealPVariant=Disabled  IVariant=InternalParameters  DVariant=InternalParameters  IntegratorVariant=Continuous  SatVariant=Disabled  AWVariant=Passthrough  PCopyVariant=Disabled  TRVariant=Disabled  FdbkBlocksVariant=Forward  IdealPFdbkVariant=Disabled  SatFdbkVariant=Disabled  DerivativeFilterVariant=ContFilter  NVariant=InternalParameters  NCopyVariant=Disabled  FilterICVariant=InternalICsFilter  IntegratorICVariant=InternalICs  ExternalResetVariant=Disabled  TRSumVariant=Passthrough  SumFdbkVariant=Disabled  SumVariant=Sum_PID  TsampFilterVariant=InternalTs  TsampNgainVariant=Passthrough  TsampIntegralVariant=Disabled_SignalSpec  ExternalSaturationOutDataTypeStr=Inherit: Same as second input  DerivativeSourceVariant=ErrorSignal  PreIntVariant=InternalPreInt
  PWM Generator (DC-DC)2 : spsPWMGeneratorDCDCLib/PWM Generator (DC-DC)  Fsw=5000  Ts=0
  PWM Generator (DC-DC)3 : spsPWMGeneratorDCDCLib/PWM Generator (DC-DC)  Fsw=5000  Ts=0
  Series RLC Branch1 : spsSeriesRLCBranchLib/Series RLC Branch  LConnTagsString=__new0  RConnTagsString=__new0  BranchType=L  Resistance=1  Inductance=1e-3  SetiL0=off  InitialCurrent=0  Capacitance=1e-6  Setx0=off  InitialVoltage=0  Measurements=None
  Series RLC Branch{2..3,5..6} (4 alike) : spsSeriesRLCBranchLib/Series RLC Branch  LConnTagsString=__new0  RConnTagsString=__new0  BranchType=RC  Resistance=0.0001  Inductance=1e-3  SetiL0=off  InitialCurrent=0  Capacitance=1000e-6  Setx0=off  InitialVoltage=0  Measurements=None
  Series RLC Branch4 : spsSeriesRLCBranchLib/Series RLC Branch  LConnTagsString=__new0  RConnTagsString=__new0  BranchType=L  Resistance=100e3  Inductance=1e-3  SetiL0=off  InitialCurrent=0  Capacitance=1e-6  Setx0=off  InitialVoltage=0  Measurements=None
  Voltage Measurement{,1..3} (4 alike) : spsVoltageMeasurementLib/Voltage Measurement  PhasorSimulation=off  OutputType=Complex  PSBequivalent=0
  disch_out + : PMIOPort  Side=Left
  disch_out - : PMIOPort  Port=2  Side=Left
  charge_in+ : PMIOPort  Port=3  Side=Left
  charge_in- : PMIOPort  Port=4  Side=Left
  disch_in+ : PMIOPort  Port=5  Side=Right
  disch_in- : PMIOPort  Port=6  Side=Right
  charge_out+ : PMIOPort  Port=7  Side=Right
  charge_out- : PMIOPort  Port=8  Side=Right
  tag scope: V1=global, V2=global
  wires:
  Voltage Measurement1/1 -> [V2]
  Voltage Measurement/1 -> [V1]
  PWM Generator (DC-DC)2/1 -> [m11]
  [V11] -> Add4/2
  Add3/1 -> PID Controller3/1
  Voltage Measurement3/1 -> [V12]
  PID Controller4/1 -> PWM Generator (DC-DC)3/1
  PID Controller3/1 -> PWM Generator (DC-DC)2/1
  Add4/1 -> PID Controller4/1
  [m11] -> Mosfet3/1
  Voltage Measurement2/1 -> [V11]
  PWM Generator (DC-DC)3/1 -> [m12]
  [m12] -> Mosfet2/1
  Constant3/1 -> Add4/1
  Constant2/1 -> Add3/1
  [V12] -> Add3/2
  [m1] -> Mosfet1/1
  [m2] -> Mosfet/1
  connections:
  Series RLC Branch5/RConn1 -- charge_in-/RConn1 -- charge_out-/RConn1 -- Voltage Measurement3/LConn2 -- Series RLC Branch6/RConn1 -- Mosfet3/RConn1 -- Voltage Measurement2/LConn2
  Mosfet1/RConn1 -- disch_in-/RConn1 -- Voltage Measurement1/LConn2 -- Series RLC Branch3/RConn1 -- disch_out -/RConn1 -- Voltage Measurement/LConn2 -- Series RLC Branch2/RConn1
  Mosfet/LConn1 -- disch_in+/RConn1 -- Voltage Measurement1/LConn1 -- Series RLC Branch3/LConn1
  Series RLC Branch4/LConn1 -- charge_in+/RConn1 -- Voltage Measurement2/LConn1 -- Series RLC Branch5/LConn1
  Series RLC Branch1/LConn1 -- Voltage Measurement/LConn1 -- Series RLC Branch2/LConn1 -- disch_out +/RConn1
  Series RLC Branch6/LConn1 -- Voltage Measurement3/LConn1 -- charge_out+/RConn1 -- Mosfet2/LConn1
  Mosfet1/LConn1 -- Series RLC Branch1/RConn1 -- Mosfet/RConn1
  Series RLC Branch4/RConn1 -- Mosfet3/LConn1 -- Mosfet2/RConn1

== system BMS/Grid1/Wall charger Connection Box/Connection Control ==
  Control : Inport
  Ideal Switch{,1..5} (6 alike) : spsIdealSwitchLib/Ideal Switch  Ron=0.001  Lon=0  IC=0  Rs=1e5  Cs=inf  Measurements=off
  NOT : Logic  Operator=NOT  IconShape=distinctive  AllPortsSameDT=off  OutDataTypeStr=boolean
  Grid R : PMIOPort  Side=Left
  Grid Y : PMIOPort  Port=2  Side=Left
  Grid B : PMIOPort  Port=3  Side=Left
  Discharge R : PMIOPort  Port=4  Side=Right
  Discharge Y : PMIOPort  Port=5  Side=Right
  Discharge B : PMIOPort  Port=6  Side=Right
  charge R : PMIOPort  Port=7  Side=Right
  charge Y : PMIOPort  Port=8  Side=Right
  charge B : PMIOPort  Port=9  Side=Right
  wires:
  Control/1 -> NOT/1, Ideal Switch2/1, Ideal Switch1/1, Ideal Switch/1
  NOT/1 -> Ideal Switch5/1, Ideal Switch4/1, Ideal Switch3/1
  connections:
  Ideal Switch2/RConn1 -- Grid B/RConn1 -- Ideal Switch5/RConn1
  Discharge R/RConn1 -- Ideal Switch/LConn1
  Discharge B/RConn1 -- Ideal Switch2/LConn1
  Ideal Switch/RConn1 -- Grid R/RConn1 -- Ideal Switch3/RConn1
  Ideal Switch1/RConn1 -- Grid Y/RConn1 -- Ideal Switch4/RConn1
  Ideal Switch4/LConn1 -- charge Y/RConn1
  Discharge Y/RConn1 -- Ideal Switch1/LConn1
  charge R/RConn1 -- Ideal Switch3/LConn1
  Ideal Switch5/LConn1 -- charge B/RConn1

== system BMS/Grid1/Wall charger Connection Box/DC-AC // AC-DC Converter ==
  Controller : Subsystem
  Measurement1 : spsThreePhaseVIMeasurementLib/Three-Phase V-I Measurement  VoltageMeasurement=phase-to-ground  SetLabelV=on  LabelV=Vabc_inv  Vpu=off  VpuLL=off  CurrentMeasurement=yes  SetLabelI=on  LabelI=Iabc_inv  Ipu=off  Pbase=100e6  Vbase=500e3  OutputType=Complex  PhasorSimulation=off  PSBequivalent=0
  PWM Generator (2-Level) : spsPWMGenerator2LevelLib/PWM Generator (2-Level)  ModulatorType=Three-phase bridge (6 pulses)  ModulatorMode=Unsynchronized  Fc=4950  Pc=90  nF=27  MinMax="[ -1  1 ]"  SamplingTechnique=Natural  ModulatingSignals=off  m=0.8  Freq=60  Phase=0  Ts=2.02e-6  ShowCarrierOutport=off
  Parallel Connection control : Constant
  Series RLC Branch2 : spsSeriesRLCBranchLib/Series RLC Branch  LConnTagsString=__new0  RConnTagsString=__new0  BranchType=RC  Resistance=10e3  Inductance=1e-3  SetiL0=off  InitialCurrent=0  Capacitance=1000e-6  Setx0=off  InitialVoltage=0  Measurements=None
  Three-Phase Series RLC Branch : spsThreePhaseSeriesRLCBranchLib/Three-Phase Series RLC Branch  LConnTagsString=A|B|C  RConnTagsString=A|B|C  BranchType=RL  Resistance=0.004332  Inductance=0.0013789184  Capacitance=1e-6  Measurements=None
  Three-Phase Breaker : spsThreePhaseBreakerLib/Three-Phase Breaker  InitialState=open  SwitchA=on  SwitchB=on  SwitchC=on  SwitchTimes="[1/60  5/60]"  External=on  BreakerResistance=0.01  SnubberResistance=1e6  SnubberCapacitance=inf  Measurements=None
  Transformer near home1 : spsThreePhaseSeriesRLCLoadLib/Three-Phase Series RLC Load  LConnTagsString=A|B|C  Configuration=Delta  NominalVoltage=380  Vabc=[1e3 1e3 1e3]  Vabcp=[1e3 1e3 1e3]  NominalFrequency=50  UnbalancedPower=off  ActivePower=100  InductivePower=0  CapacitivePower=5000  Pabc=[10e3 9e3 11e3]  QLabc=[100 90 110]  QCabc=[100 90 110]  Pabcp=[10e3 9e3 11e3]  QLabcp=[100 90 110]  QCabcp=[100 90 110]  Measurements=None  LoadType=constant Z
  Universal Bridge : spsUniversalBridgeLib/Universal Bridge  Arms=3  SnubberResistance=1e5  SnubberCapacitance=inf  Device=IGBT / Diodes  Ron=1e-3  Lon=0  ForwardVoltages="[  0  0  ]"  ForwardVoltage=0  GTOparameters=[ 10e-6 , 20e-6 ]  IGBTparameters=[ 1e-6 , 2e-6 ]  Measurements=None  Measurements_2=None  converterType=Rectifier
  Universal Bridge1 : spsUniversalBridgeLib/Universal Bridge  Arms=3  SnubberResistance=1e5  SnubberCapacitance=inf  Device=Diodes  Ron=1e-3  Lon=0  ForwardVoltages="[  0  0  ]"  ForwardVoltage=0  GTOparameters=[ 10e-6 , 20e-6 ]  IGBTparameters=[ 1e-6 , 2e-6 ]  Measurements=None  Measurements_2=None  converterType=Rectifier
  Discharge_R : PMIOPort  Side=Left
  Discharge_Y : PMIOPort  Port=2  Side=Left
  Discharge_B : PMIOPort  Port=3  Side=Left
  charge_R : PMIOPort  Port=4  Side=Left
  charge_Y : PMIOPort  Port=5  Side=Left
  charge_B : PMIOPort  Port=6  Side=Left
  Discharge + : PMIOPort  Port=7  Side=Right
  Discharge - : PMIOPort  Port=8  Side=Right
  charge+ : PMIOPort  Port=9  Side=Right
  charge- : PMIOPort  Port=10  Side=Right
  wires:
  PWM Generator (2-Level)/1 -> Universal Bridge/1
  Parallel Connection control/1 -> Three-Phase Breaker/1
  [ref] -> PWM Generator (2-Level)/1
  connections:
  Universal Bridge1/LConn2 -- charge_Y/RConn1
  Universal Bridge1/LConn3 -- charge_B/RConn1
  Discharge_Y/RConn1 -- Three-Phase Breaker/RConn2
  Three-Phase Series RLC Branch/RConn1 -- Transformer near home1/LConn1 -- Measurement1/LConn1
  Measurement1/RConn2 -- Three-Phase Breaker/LConn2
  charge-/RConn1 -- Series RLC Branch2/RConn1 -- Universal Bridge1/RConn2
  Three-Phase Series RLC Branch/RConn3 -- Measurement1/LConn3 -- Transformer near home1/LConn3
  Discharge_B/RConn1 -- Three-Phase Breaker/RConn3
  Three-Phase Series RLC Branch/LConn2 -- Universal Bridge/LConn2
  Universal Bridge/LConn1 -- Three-Phase Series RLC Branch/LConn1
  Discharge -/RConn1 -- Universal Bridge/RConn2
  Universal Bridge/LConn3 -- Three-Phase Series RLC Branch/LConn3
  Three-Phase Series RLC Branch/RConn2 -- Measurement1/LConn2 -- Transformer near home1/LConn2
  Discharge +/RConn1 -- Universal Bridge/RConn1
  charge+/RConn1 -- Series RLC Branch2/LConn1 -- Universal Bridge1/RConn1
  Discharge_R/RConn1 -- Three-Phase Breaker/RConn1
  Measurement1/RConn1 -- Three-Phase Breaker/LConn1
  Measurement1/RConn3 -- Three-Phase Breaker/LConn3
  Universal Bridge1/LConn1 -- charge_R/RConn1
